simulink library "TestLib_HV_Manager"  (Simulink 7.5)
settings: Solver=ode1  StartTime=0.0  StopTime=Inf  FixedStep=0.001  RelTol=1e-3
PostLoadFcn:
  | , if any(exist('dsrtsu_mdlpostloadfcn', 'file') == [2, 3, 6]), try dsrtsu_mdlpostloadfcn('Execute', bdroot); catch fprintf('Error in PostLoadFcn (dsrtsu_mdlpostloadfcn) for model "%s":\n %s\n', bdroot, lasterr); end, end,
undefined symbols (not defined in the file): cal
libraries: EC2_libraries x13, simulink x9, TestLib_BCM_Manager x1
settings Model: DSRTSU_INTERNAL_RTI_VER=380  DSRTSU_INTERNAL_RTI_TYPE=rti1006  RTICANMMDATA=struct('GeneralSetupData',struct('modelroot',['C:\Users\EC2user\Documents\SVN__Controls\ecocar2_Controls\PTTR Alpha Branch\Libraries\CAN'],'generalsettings',struct('filesettings',struct('destfolder',struct('Name','RTICANMM_FILES','Check',1),'buildfolder',struct('Name','.','Check',1),'AbsDestfolder',struct('Name',['C:\Users\EC2user\Documents\SVN__Controls\ecocar2_Controls\PTTR Alpha Branch\Libraries\Diagnostics\Testing\RTICANMM_FILES']),'AbsBuildfolder',struct('Name',['C:\Users\EC2user\Documents\SVN__Controls\ecocar2_Controls\PTTR Alpha Branch\Libraries\CAN']))),'options',struct('addpaths',1,'rmpaths',1,'addtrcexclusion',logical(1),'cannavigator',struct('checkmonitoring',0,'serviceno','31','hostservicedefheader',struct('name','x','path','x')),'show_usrtrc',0,'use_usrtrc',0),'advanced',struct('options',[1 1 1 1 1 1 1 1 1 1 1 1 1 1 1 1 1 1 1 1 1 1 1 1 1 1 1 1 1 1 1 1 1 1 1 1 1 1 1 1 1 1 1 1 1 1 1 1 1 1 1 1 1 1 1 1 1 1 1 1 1 1 1 1 1 1 1 1 1 1 1 1 1 1 1 1 1 1 1 1 1 1 1 1 1 1 1 1 1 1 1 1 1 1 1 1 1 1 1 1]),'MPSetup',{{}},'modelname','DIAG_CAN_OUT','block','TestLib_HV_Manager'))  Creator=idan  LastModifiedBy=Yuxia^_^

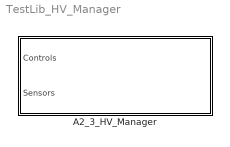
== system TestLib_HV_Manager ==
  A2_3_HV_Manager : Subsystem

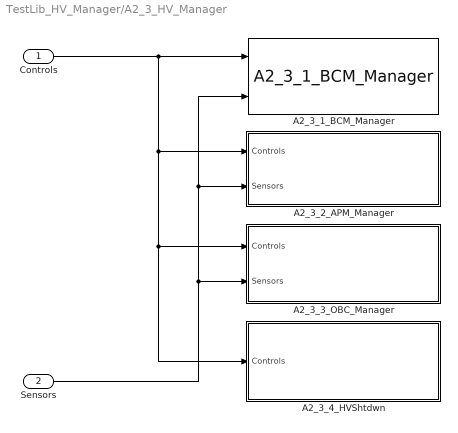
== system TestLib_HV_Manager/A2_3_HV_Manager ==
  Controls : Inport  OutDataType=fixdt(1, 16)  OutScaling=2^0
  Sensors : Inport  Port=2  OutDataType=fixdt(1, 16)  OutScaling=2^0
  A2_3_1_BCM_Manager : TestLib_BCM_Manager/A2_3_1_BCM_Manager  SystemSampleTime=-1
  A2_3_2_APM_Manager : Subsystem
  A2_3_3_OBC_Manager : Subsystem
  A2_3_4_HVShtdwn : Subsystem
  wires:
  Sensors/1 -> A2_3_3_OBC_Manager/2(Sensors), A2_3_1_BCM_Manager/2, A2_3_2_APM_Manager/2(Sensors)
  Controls/1 -> A2_3_1_BCM_Manager/1, A2_3_2_APM_Manager/1(Controls), A2_3_3_OBC_Manager/1(Controls), A2_3_4_HVShtdwn/1(Controls)

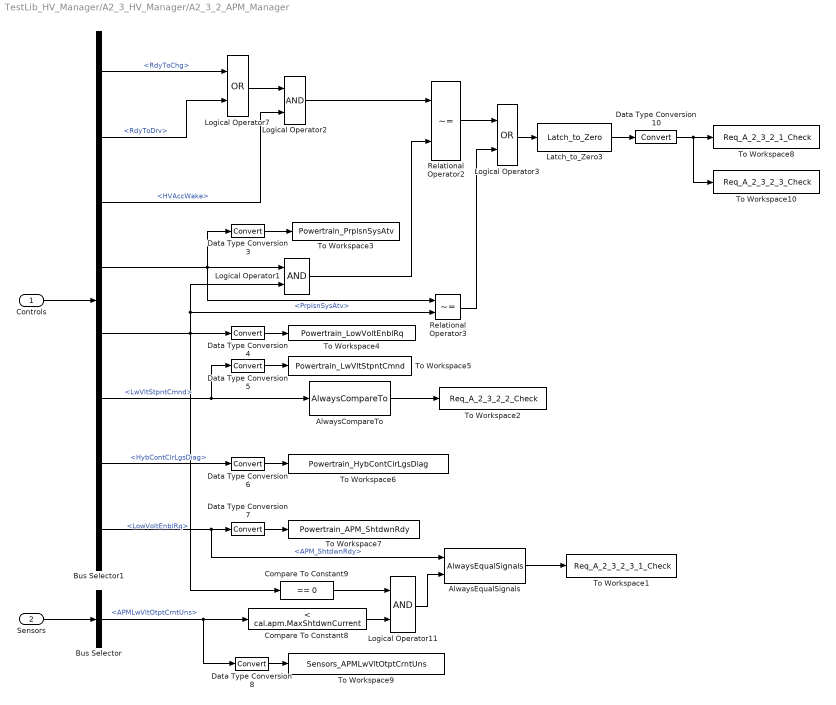
== system TestLib_HV_Manager/A2_3_HV_Manager/A2_3_2_APM_Manager ==
  Controls : Inport  OutDataType=fixdt(1, 16)  OutScaling=2^0
  Sensors : Inport  Port=2  OutDataType=fixdt(1, 16)  OutScaling=2^0
  AlwaysCompareTo : EC2_libraries/AlwaysCompareTo  SystemSampleTime=-1  exp_val=cal.apm.LowVoltageSetpoint
  AlwaysEqualSignals : EC2_libraries/AlwaysEqualSignals  SystemSampleTime=-1
  Bus Selector : BusSelector  OutputSignals=Sensors_CAN.APM_HS_Tx.Accessory_Pwr_Mod_Gen_Status_1.APMLwVltOtptCrntUns
  Bus Selector1 : BusSelector  OutputSignals=Powertrain_SC_Controls.HV_Status.RdyToChg,Powertrain_SC_Controls.HV_Status.RdyToDrv,Powertrain_SC_Controls.HV_Status.HVAccWake,Powertrain_SC_Controls.APM_Controls.PrplsnSysAtv,Powertrain_SC_Controls.APM_Controls.LowVoltEnblRq,Powertrain_SC_Controls.APM_Controls.LwVltStpntCmnd,Powertrain_SC_Controls.APM_Controls.HybContClrLgsDiag,Powertrain_SC_Controls.APM_Status.APM_ShtdwnRdy
  Compare To Constant8 : simulink/Logic and Bit Operations/Compare To Constant  SystemSampleTime=-1  relop=<  const=cal.apm.MaxShtdwnCurrent  LogicOutDataTypeMode=uint8
  Compare To Constant9 : simulink/Logic and Bit Operations/Compare To Constant  SystemSampleTime=-1  relop===  const=0  LogicOutDataTypeMode=boolean
  Data Type Conversion{3..8,10} (7 alike) : DataTypeConversion  OutDataType=fixdt(1, 16)  OutScaling=2^0
  Latch_to_Zero3 : EC2_libraries/Latch_to_Zero  SystemSampleTime=-1
  Logical Operator1 : Logic  AllPortsSameDT=off  OutDataTypeMode=boolean  OutDataTypeStr=boolean
  Logical Operator11 : Logic  AllPortsSameDT=off  OutDataTypeMode=boolean  OutDataTypeStr=boolean
  Logical Operator2 : Logic  AllPortsSameDT=off  OutDataTypeMode=boolean  OutDataTypeStr=boolean
  Logical Operator3 : Logic  Operator=OR  AllPortsSameDT=off  OutDataTypeMode=boolean  OutDataTypeStr=boolean
  Logical Operator7 : Logic  Operator=OR  AllPortsSameDT=off  OutDataTypeMode=boolean  OutDataTypeStr=boolean
  Relational Operator2 : RelationalOperator  Operator=~=  LogicOutDataTypeMode=boolean  LogicDataType=fixdt(0, 8)  OutDataTypeStr=boolean
  Relational Operator3 : RelationalOperator  Operator=~=  LogicOutDataTypeMode=boolean  LogicDataType=fixdt(0, 8)  OutDataTypeStr=boolean
  To Workspace1 : ToWorkspace  VariableName=Req_A_2_3_2_3_1_Check  SampleTime=-1  SaveFormat=Array
      settings: Decimation=WORKSPACE_DECIMATION
  To Workspace10 : ToWorkspace  VariableName=Req_A_2_3_2_3_Check  SampleTime=-1  SaveFormat=Array
      settings: Decimation=WORKSPACE_DECIMATION
  To Workspace2 : ToWorkspace  VariableName=Req_A_2_3_2_2_Check  SampleTime=-1  SaveFormat=Array
      settings: Decimation=WORKSPACE_DECIMATION
  To Workspace3 : ToWorkspace  VariableName=Powertrain_PrplsnSysAtv  SampleTime=-1  SaveFormat=Array
      settings: Decimation=WORKSPACE_DECIMATION
  To Workspace4 : ToWorkspace  VariableName=Powertrain_LowVoltEnblRq  SampleTime=-1  SaveFormat=Array
      settings: Decimation=WORKSPACE_DECIMATION
  To Workspace5 : ToWorkspace  VariableName=Powertrain_LwVltStpntCmnd  SampleTime=-1  SaveFormat=Array
      settings: Decimation=WORKSPACE_DECIMATION
  To Workspace6 : ToWorkspace  VariableName=Powertrain_HybContClrLgsDiag  SampleTime=-1  SaveFormat=Array
      settings: Decimation=WORKSPACE_DECIMATION
  To Workspace7 : ToWorkspace  VariableName=Powertrain_APM_ShtdwnRdy  SampleTime=-1  SaveFormat=Array
      settings: Decimation=WORKSPACE_DECIMATION
  To Workspace8 : ToWorkspace  VariableName=Req_A_2_3_2_1_Check  SampleTime=-1  SaveFormat=Array
      settings: Decimation=WORKSPACE_DECIMATION
  To Workspace9 : ToWorkspace  VariableName=Sensors_APMLwVltOtptCrntUns  SampleTime=-1  SaveFormat=Array
      settings: Decimation=WORKSPACE_DECIMATION
  wires:
  AlwaysEqualSignals/1 -> To Workspace1/1
  Logical Operator3/1 -> Latch_to_Zero3/1
  Relational Operator3/1 -> Logical Operator3/2
  Relational Operator2/1 -> Logical Operator3/1
  Logical Operator2/1 -> Relational Operator2/1
  Bus Selector1/3 -> Logical Operator2/2  "<HVAccWake>"
  Logical Operator1/1 -> Relational Operator2/2
  Data Type Conversion10/1 -> To Workspace8/1, To Workspace10/1
  Latch_to_Zero3/1 -> Data Type Conversion10/1
  Logical Operator7/1 -> Logical Operator2/1
  AlwaysCompareTo/1 -> To Workspace2/1
  Logical Operator11/1 -> AlwaysEqualSignals/2
  Compare To Constant8/1 -> Logical Operator11/2
  Compare To Constant9/1 -> Logical Operator11/1
  Data Type Conversion7/1 -> To Workspace7/1
  Data Type Conversion6/1 -> To Workspace6/1
  Data Type Conversion5/1 -> To Workspace5/1
  Data Type Conversion4/1 -> To Workspace4/1
  Data Type Conversion3/1 -> To Workspace3/1
  Bus Selector1/8 -> AlwaysEqualSignals/1, Data Type Conversion7/1  "<APM_ShtdwnRdy>"
  Bus Selector1/7 -> Data Type Conversion6/1  "<HybContClrLgsDiag>"
  Bus Selector1/6 -> AlwaysCompareTo/1, Data Type Conversion5/1  "<LwVltStpntCmnd>"
  Bus Selector1/5 -> Relational Operator3/2, Logical Operator1/2, Compare To Constant9/1, Data Type Conversion4/1  "<LowVoltEnblRq>"
  Bus Selector1/4 -> Relational Operator3/1, Logical Operator1/1, Data Type Conversion3/1  "<PrplsnSysAtv>"
  Bus Selector1/2 -> Logical Operator7/2  "<RdyToDrv>"
  Bus Selector1/1 -> Logical Operator7/1  "<RdyToChg>"
  Data Type Conversion8/1 -> To Workspace9/1
  Bus Selector/1 -> Compare To Constant8/1, Data Type Conversion8/1  "<APMLwVltOtptCrntUns>"
  Controls/1 -> Bus Selector1/1
  Sensors/1 -> Bus Selector/1

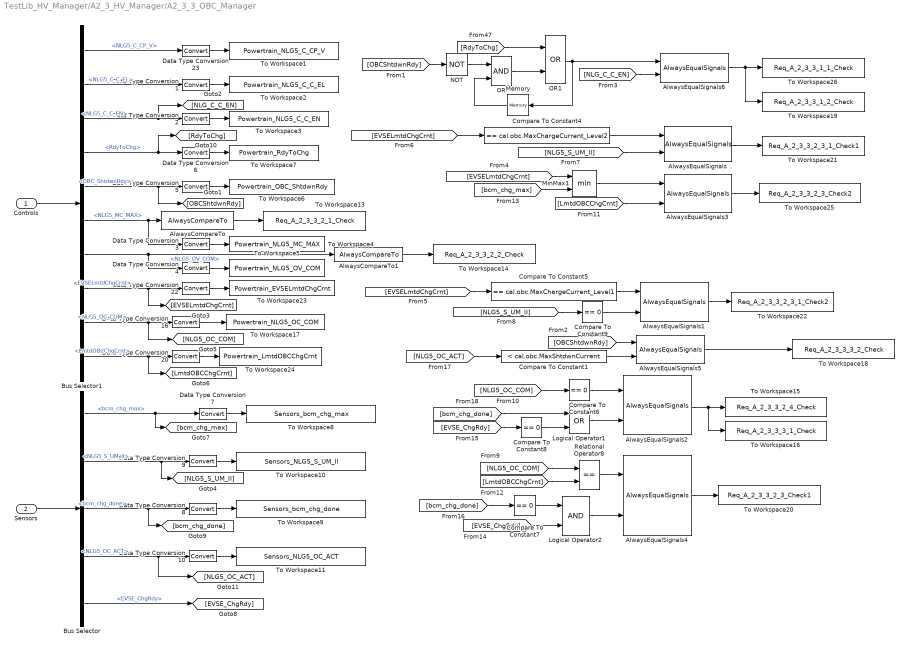
== system TestLib_HV_Manager/A2_3_HV_Manager/A2_3_3_OBC_Manager ==
  Controls : Inport  OutDataType=fixdt(1, 16)  OutScaling=2^0
  Sensors : Inport  Port=2  OutDataType=fixdt(1, 16)  OutScaling=2^0
  AlwaysCompareTo : EC2_libraries/AlwaysCompareTo  SystemSampleTime=-1  exp_val=cal.obc.MaxMainsCurrent
  AlwaysCompareTo1 : EC2_libraries/AlwaysCompareTo  SystemSampleTime=-1  exp_val=cal.obc.MaxOutputVoltage
  AlwaysEqualSignals{,1..6} (7 alike) : EC2_libraries/AlwaysEqualSignals  SystemSampleTime=-1
  Bus Selector : BusSelector  OutputSignals=Sensors_CAN.BCM_HS_Tx.BCM_Limits.bcm_chg_max,Sensors_CAN.OBC_HS_Tx.NLG5_ST.NLG5_S_UM_II,Sensors_CAN.BCM_HS_Tx.BCM_Status.bcm_chg_done,Sensors_CAN.OBC_HS_Tx.NLG5_ACT_I.NLG5_OC_ACT,Analog.EVSE_ChgRdy
  Bus Selector1 : BusSelector  OutputSignals=Powertrain_SC_Controls.OBC_Controls.NLG5_C_CP_V,Powertrain_SC_Controls.OBC_Controls.NLG5_C_C_EL,Powertrain_SC_Controls.OBC_Controls.NLG5_C_C_EN,Powertrain_SC_Controls.HV_Status.RdyToChg,Powertrain_SC_Controls.OBC_Status.OBC_ShtdwnRdy,Powertrain_SC_Controls.OBC_Controls.NLG5_MC_MAX,Powertrain_SC_Controls.OBC_Controls.NLG5_OV_COM,Powertrain_SC_Controls.OBC_Status.EVSELmtdChgCrnt,Powertrain_SC_Controls.OBC_Controls.NLG5_OC_COM,Powertrain_SC_Controls.OBC_Status.LmtdOBCChgCrnt
  Compare To Constant1 : simulink/Logic and Bit Operations/Compare To Constant  SystemSampleTime=-1  relop=<  const=cal.obc.MaxShtdwnCurrent  LogicOutDataTypeMode=boolean
  Compare To Constant4 : simulink/Logic and Bit Operations/Compare To Constant  SystemSampleTime=-1  relop===  const=cal.obc.MaxChargeCurrent_Level2  LogicOutDataTypeMode=boolean
  Compare To Constant5 : simulink/Logic and Bit Operations/Compare To Constant  SystemSampleTime=-1  relop===  const=cal.obc.MaxChargeCurrent_Level1  LogicOutDataTypeMode=boolean
  Compare To Constant{6..9} (4 alike) : simulink/Logic and Bit Operations/Compare To Constant  SystemSampleTime=-1  relop===  const=0  LogicOutDataTypeMode=boolean
  Data Type Conversion{1..10,16,20,22..23} (14 alike) : DataTypeConversion  OutDataType=fixdt(1, 16)  OutScaling=2^0
  Logical Operator1 : Logic  Operator=OR  AllPortsSameDT=off  OutDataTypeMode=boolean  OutDataTypeStr=boolean
  Logical Operator2 : Logic  AllPortsSameDT=off  OutDataTypeMode=boolean  OutDataTypeStr=boolean
  Memory : Memory
  MinMax1 : MinMax  Inputs=2
  NOT : Logic  Operator=NOT  OutDataTypeMode=boolean  OutDataTypeStr=boolean
  OR : Logic  OutDataTypeMode=boolean  OutDataTypeStr=boolean
  OR1 : Logic  Operator=OR  OutDataTypeMode=boolean  OutDataTypeStr=boolean
  Relational Operator8 : RelationalOperator  Operator===  LogicOutDataTypeMode=boolean  LogicDataType=fixdt(0, 8)  OutDataTypeStr=boolean
  To Workspace1 : ToWorkspace  VariableName=Powertrain_NLG5_C_CP_V  SampleTime=-1  SaveFormat=Array
      settings: Decimation=WORKSPACE_DECIMATION
  To Workspace10 : ToWorkspace  VariableName=Sensors_NLG5_S_UM_II  SampleTime=-1  SaveFormat=Array
      settings: Decimation=WORKSPACE_DECIMATION
  To Workspace11 : ToWorkspace  VariableName=Sensors_NLG5_OC_ACT  SampleTime=-1  SaveFormat=Array
      settings: Decimation=WORKSPACE_DECIMATION
  To Workspace13 : ToWorkspace  VariableName=Req_A_2_3_3_2_1_Check  SampleTime=-1  SaveFormat=Array
      settings: Decimation=WORKSPACE_DECIMATION
  To Workspace14 : ToWorkspace  VariableName=Req_A_2_3_3_2_2_Check  SampleTime=-1  SaveFormat=Array
      settings: Decimation=WORKSPACE_DECIMATION
  To Workspace15 : ToWorkspace  VariableName=Req_A_2_3_3_2_4_Check  SampleTime=-1  SaveFormat=Array
      settings: Decimation=WORKSPACE_DECIMATION
  To Workspace16 : ToWorkspace  VariableName=Req_A_2_3_3_3_1_Check  SampleTime=-1  SaveFormat=Array
      settings: Decimation=WORKSPACE_DECIMATION
  To Workspace17 : ToWorkspace  VariableName=Powertrain_NLG5_OC_COM  SampleTime=-1  SaveFormat=Array
      settings: Decimation=WORKSPACE_DECIMATION
  To Workspace18 : ToWorkspace  VariableName=Req_A_2_3_3_3_2_Check  SampleTime=-1  SaveFormat=Array
      settings: Decimation=WORKSPACE_DECIMATION
  To Workspace19 : ToWorkspace  VariableName=Req_A_2_3_3_1_2_Check  SampleTime=-1  SaveFormat=Array
      settings: Decimation=WORKSPACE_DECIMATION
  To Workspace2 : ToWorkspace  VariableName=Powertrain_NLG5_C_C_EL  SampleTime=-1  SaveFormat=Array
      settings: Decimation=WORKSPACE_DECIMATION
  To Workspace20 : ToWorkspace  VariableName=Req_A_2_3_3_2_3_Check1  SampleTime=-1  SaveFormat=Array
      settings: Decimation=WORKSPACE_DECIMATION
  To Workspace21 : ToWorkspace  VariableName=Req_A_2_3_3_2_3_1_Check1  SampleTime=-1  SaveFormat=Array
      settings: Decimation=WORKSPACE_DECIMATION
  To Workspace22 : ToWorkspace  VariableName=Req_A_2_3_3_2_3_1_Check2  SampleTime=-1  SaveFormat=Array
      settings: Decimation=WORKSPACE_DECIMATION
  To Workspace23 : ToWorkspace  VariableName=Powertrain_EVSELmtdChgCrnt  SampleTime=-1  SaveFormat=Array
      settings: Decimation=WORKSPACE_DECIMATION
  To Workspace24 : ToWorkspace  VariableName=Powertrain_LmtdOBCChgCrnt  SampleTime=-1  SaveFormat=Array
      settings: Decimation=WORKSPACE_DECIMATION
  To Workspace25 : ToWorkspace  VariableName=Req_A_2_3_3_2_3_Check2  SampleTime=-1  SaveFormat=Array
      settings: Decimation=WORKSPACE_DECIMATION
  To Workspace26 : ToWorkspace  VariableName=Req_A_2_3_3_1_1_Check  SampleTime=-1  SaveFormat=Array
      settings: Decimation=WORKSPACE_DECIMATION
  To Workspace3 : ToWorkspace  VariableName=Powertrain_NLG5_C_C_EN  SampleTime=-1  SaveFormat=Array
      settings: Decimation=WORKSPACE_DECIMATION
  To Workspace4 : ToWorkspace  VariableName=Powertrain_NLG5_MC_MAX  SampleTime=-1  SaveFormat=Array
      settings: Decimation=WORKSPACE_DECIMATION
  To Workspace5 : ToWorkspace  VariableName=Powertrain_NLG5_OV_COM  SampleTime=-1  SaveFormat=Array
      settings: Decimation=WORKSPACE_DECIMATION
  To Workspace6 : ToWorkspace  VariableName=Powertrain_OBC_ShtdwnRdy  SampleTime=-1  SaveFormat=Array
      settings: Decimation=WORKSPACE_DECIMATION
  To Workspace7 : ToWorkspace  VariableName=Powertrain_RdyToChg  SampleTime=-1  SaveFormat=Array
      settings: Decimation=WORKSPACE_DECIMATION
  To Workspace8 : ToWorkspace  VariableName=Sensors_bcm_chg_max  SampleTime=-1  SaveFormat=Array
      settings: Decimation=WORKSPACE_DECIMATION
  To Workspace9 : ToWorkspace  VariableName=Sensors_bcm_chg_done  SampleTime=-1  SaveFormat=Array
      settings: Decimation=WORKSPACE_DECIMATION
  wires:
  Relational Operator8/1 -> AlwaysEqualSignals4/1
  AlwaysEqualSignals3/1 -> To Workspace25/1
  AlwaysEqualSignals4/1 -> To Workspace20/1
  Logical Operator2/1 -> AlwaysEqualSignals4/2
  Compare To Constant7/1 -> Logical Operator2/1
  MinMax1/1 -> AlwaysEqualSignals3/1
  Compare To Constant9/1 -> AlwaysEqualSignals1/2
  Bus Selector1/8 -> Data Type Conversion22/1, [EVSELmtdChgCrnt]  "<EVSELmtdChgCrnt>"
  Bus Selector1/10 -> Data Type Conversion20/1, [LmtdOBCChgCrnt]  "<LmtdOBCChgCrnt>"
  Data Type Conversion22/1 -> To Workspace23/1
  Data Type Conversion20/1 -> To Workspace24/1
  AlwaysEqualSignals1/1 -> To Workspace22/1
  Logical Operator1/1 -> AlwaysEqualSignals2/2
  AlwaysEqualSignals/1 -> To Workspace21/1
  Memory/1 -> OR/2
  NOT/1 -> OR/1
  OR1/1 -> Memory/1, AlwaysEqualSignals6/1
  OR/1 -> OR1/2
  AlwaysEqualSignals6/1 -> To Workspace19/1, To Workspace26/1
  AlwaysEqualSignals5/1 -> To Workspace18/1
  Compare To Constant8/1 -> Logical Operator1/2
  AlwaysEqualSignals2/1 -> To Workspace16/1, To Workspace15/1
  AlwaysCompareTo1/1 -> To Workspace14/1
  AlwaysCompareTo/1 -> To Workspace13/1
  Compare To Constant1/1 -> AlwaysEqualSignals5/2
  Compare To Constant6/1 -> AlwaysEqualSignals2/1
  Compare To Constant5/1 -> AlwaysEqualSignals1/1
  Compare To Constant4/1 -> AlwaysEqualSignals/1
  Bus Selector1/9 -> Data Type Conversion16/1, [NLG5_OC_COM]  "<NLG5_OC_COM>"
  Data Type Conversion16/1 -> To Workspace17/1
  Bus Selector/5 -> [EVSE_ChgRdy]  "<EVSE_ChgRdy>"
  Bus Selector/4 -> Data Type Conversion10/1, [NLG5_OC_ACT]  "<NLG5_OC_ACT>"
  Bus Selector/2 -> Data Type Conversion9/1, [NLG5_S_UM_II]  "<NLG5_S_UM_II>"
  Bus Selector/1 -> Data Type Conversion7/1, [bcm_chg_max]  "<bcm_chg_max>"
  Bus Selector/3 -> Data Type Conversion8/1, [bcm_chg_done]  "<bcm_chg_done>"
  Data Type Conversion10/1 -> To Workspace11/1
  Data Type Conversion9/1 -> To Workspace10/1
  Data Type Conversion7/1 -> To Workspace8/1
  Bus Selector1/4 -> Data Type Conversion6/1, [RdyToChg]  "<RdyToChg>"
  Bus Selector1/5 -> Data Type Conversion5/1, [OBCShtdwnRdy]  "<OBC_ShtdwnRdy>"
  Bus Selector1/7 -> Data Type Conversion4/1, AlwaysCompareTo1/1  "<NLG5_OV_COM>"
  Bus Selector1/6 -> Data Type Conversion3/1, AlwaysCompareTo/1  "<NLG5_MC_MAX>"
  Bus Selector1/3 -> Data Type Conversion2/1, [NLG_C_C_EN]  "<NLG5_C_C_EN>"
  Bus Selector1/2 -> Data Type Conversion1/1  "<NLG5_C_C_EL>"
  Bus Selector1/1 -> Data Type Conversion23/1  "<NLG5_C_CP_V>"
  Data Type Conversion6/1 -> To Workspace7/1
  Data Type Conversion5/1 -> To Workspace6/1
  Data Type Conversion4/1 -> To Workspace5/1
  Data Type Conversion3/1 -> To Workspace4/1
  Data Type Conversion2/1 -> To Workspace3/1
  Data Type Conversion1/1 -> To Workspace2/1
  Data Type Conversion8/1 -> To Workspace9/1
  Data Type Conversion23/1 -> To Workspace1/1
  Controls/1 -> Bus Selector1/1
  Sensors/1 -> Bus Selector/1
  [RdyToChg] -> OR1/1
  [OBCShtdwnRdy] -> NOT/1
  [OBCShtdwnRdy] -> AlwaysEqualSignals5/1
  [NLG_C_C_EN] -> AlwaysEqualSignals6/2
  [EVSELmtdChgCrnt] -> MinMax1/1
  [EVSELmtdChgCrnt] -> Compare To Constant5/1
  [EVSELmtdChgCrnt] -> Compare To Constant4/1
  [NLG5_S_UM_II] -> AlwaysEqualSignals/2
  [NLG5_S_UM_II] -> Compare To Constant9/1
  [NLG5_OC_COM] -> Relational Operator8/1
  [NLG5_OC_COM] -> Compare To Constant6/1
  [LmtdOBCChgCrnt] -> AlwaysEqualSignals3/2
  [LmtdOBCChgCrnt] -> Relational Operator8/2
  [bcm_chg_max] -> MinMax1/2
  [EVSE_ChgRdy] -> Logical Operator2/2
  [EVSE_ChgRdy] -> Compare To Constant8/1
  [bcm_chg_done] -> Compare To Constant7/1
  [NLG5_OC_ACT] -> Compare To Constant1/1
  [bcm_chg_done] -> Logical Operator1/1

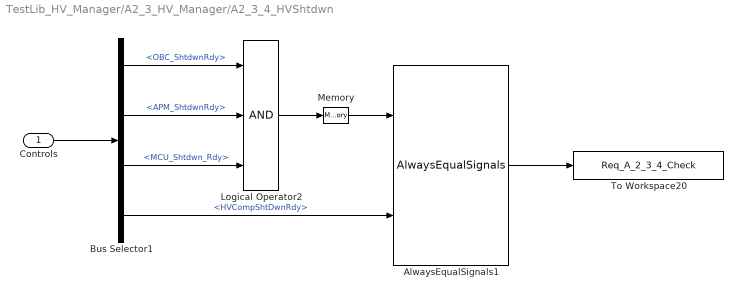
== system TestLib_HV_Manager/A2_3_HV_Manager/A2_3_4_HVShtdwn ==
  Controls : Inport  OutDataType=fixdt(1, 16)  OutScaling=2^0
  AlwaysEqualSignals1 : EC2_libraries/AlwaysEqualSignals  SystemSampleTime=-1
  Bus Selector1 : BusSelector  OutputSignals=Powertrain_SC_Controls.OBC_Status.OBC_ShtdwnRdy,Powertrain_SC_Controls.APM_Status.APM_ShtdwnRdy,Powertrain_SC_Controls.MCU_Status.MCU_Shtdwn_Rdy,Powertrain_SC_Controls.HV_Status.HVCompShtDwnRdy
  Logical Operator2 : Logic  Inputs=3  AllPortsSameDT=off  OutDataTypeMode=boolean  OutDataTypeStr=boolean
  Memory : Memory
  To Workspace20 : ToWorkspace  VariableName=Req_A_2_3_4_Check  SampleTime=-1  SaveFormat=Array
      settings: Decimation=WORKSPACE_DECIMATION
  wires:
  Bus Selector1/4 -> AlwaysEqualSignals1/2  "<HVCompShtDwnRdy>"
  Bus Selector1/3 -> Logical Operator2/3  "<MCU_Shtdwn_Rdy>"
  Logical Operator2/1 -> Memory/1
  AlwaysEqualSignals1/1 -> To Workspace20/1
  Bus Selector1/2 -> Logical Operator2/2  "<APM_ShtdwnRdy>"
  Bus Selector1/1 -> Logical Operator2/1  "<OBC_ShtdwnRdy>"
  Controls/1 -> Bus Selector1/1
  Memory/1 -> AlwaysEqualSignals1/1
